simulink model "Appl_DrMemory_CtrlModel"  (R2018b)
settings: configuration reference "CodeConfig_10_ms" (kept outside this file)
undefined symbols (not defined in the file): CAL_DrMem_100MS, CAL_DrMem_90MS, D_DRMEM_SPEED_5, D_ToleranceDistance, FALSE, TRUE
libraries: DareLib x92, simulink x1
(part 3 of 3)

== stateflow chart Appl_DrMemory_CtrlModel/UpDataInputInfo/InputSignalProcess/MemorySetCallPreconditionDeal/PreconditionDeal ==
  state MemorySetPreconditionDeal [parallel]
    settings: executionOrder=1
    state PreconditionSatisfied
      en:
      MemSetPC_Flag = TRUE;
    state PreconditionNotSatisfied
      en:
      MemSetPC_Flag = FALSE;
    (default) -> MemorySetPreconditionDeal.PreconditionNotSatisfied
    MemorySetPreconditionDeal.PreconditionNotSatisfied -> MemorySetPreconditionDeal.PreconditionSatisfied : /*调节配置 == 1six way motor ||  2 twelve way motor
        | && 记忆功能使能 == 0x1:TRUE
        | && 座椅已学习
        | && 座椅运动类型 == 0x0:enNULL
        | && 座椅霍尔故障标志位 == FALSE
        | && 座椅继电器粘连故障标志位 == FALSE
        | && 座椅堵转故障标志位 == FALSE
        | && IVI_NapMode_SwtichSet != 0x1:打开小憩模式
        | && 电压模式 == 正常
        | && DrMem_NapMode != enNapMode.EN_NapMode_Open...
        | /PreMemSetStop = 0x0:enNone;*/
        | [(DrMem_AdjustEnable == 1 || DrMem_AdjustEnable == 2) ...
        | && DrMem_MemoryConfig == TRUE ...
        | && DrMem_SeatLearnResult == TRUE ...
        | && DrMem_CurrentMoveType == enSeatMotorRunType.EN_NULL ...
        | && DrMem_AnyoneHallFaultSts == FALSE ...
        | && DrMem_AnyoneRelayFaultSts == FALSE ...
        | && DrMem_AnyoneLockFaultSts == FALSE ...
        | && DrMem_VoltSatisfy == TRUE ...
        | && DrMem_VoltMode == enFinalPowerMode.EN_NORMAL_VOLT]
        | /PreMemSetStop = enMemStopCause.EN_MemStop_NULL;
    MemorySetPreconditionDeal.PreconditionSatisfied -> MemorySetPreconditionDeal.PreconditionNotSatisfied [order 1] : /*记忆功能使能 != 0x1:TRUE
        | /PreMemCallStop = 0xA:enConfigError;*/
        | [(DrMem_AdjustEnable != 1 && DrMem_AdjustEnable != 2) || DrMem_MemoryConfig != TRUE]
        | /PreMemSetStop = enMemStopCause.EN_MemStop_ConfigError;
    MemorySetPreconditionDeal.PreconditionSatisfied -> MemorySetPreconditionDeal.PreconditionNotSatisfied [order 2] : /*!座椅已学习
        | /PreMemSetStop = 0x1:enNotLearn;*/
        | [DrMem_SeatLearnResult != TRUE]
        | /PreMemSetStop = enMemStopCause.EN_MemStop_Learn;
    MemorySetPreconditionDeal.PreconditionSatisfied -> MemorySetPreconditionDeal.PreconditionNotSatisfied [order 3] : /*座椅运动类型 != 0x0:enNULL
        | /PreMemSetStop = 0x2:enOtherMove;*/
        | [DrMem_CurrentMoveType != enSeatMotorRunType.EN_NULL]
        | /PreMemSetStop = enMemStopCause.EN_MemStop_OtherMove;
    MemorySetPreconditionDeal.PreconditionSatisfied -> MemorySetPreconditionDeal.PreconditionNotSatisfied [order 4] : /*座椅霍尔故障标志位 != FALSE
        | /PreMemSetStop = 0x3:enHallError;*/
        | [DrMem_AnyoneHallFaultSts != FALSE]
        | /PreMemSetStop = enMemStopCause.EN_MemStop_HallErr;
    MemorySetPreconditionDeal.PreconditionSatisfied -> MemorySetPreconditionDeal.PreconditionNotSatisfied [order 5] : /*座椅继电器粘连故障标志位 != FALSE
        | /PreMemSetStop = 0x4:enRelayError;*/
        | [DrMem_AnyoneRelayFaultSts != FALSE]
        | /PreMemSetStop = enMemStopCause.EN_MemStop_RelayErr;
    MemorySetPreconditionDeal.PreconditionSatisfied -> MemorySetPreconditionDeal.PreconditionNotSatisfied [commented out] : /*IVI_NapMode_SwtichSet == 0x1:打开小憩模式
        | /PreMemSetStop = 0xB:enNapError;*/
        | [DrMem_NapMode == enNapMode.EN_NapMode_Open]
        | /PreMemSetStop = enMemStopCause.EN_MemStop_NapError;
    MemorySetPreconditionDeal.PreconditionSatisfied -> MemorySetPreconditionDeal.PreconditionNotSatisfied [order 7] : /*座椅堵转故障标志位 != FALSE
        | /PreMemSetStop = 0x5:EN_MemStop_StallErr(;*/
        | [DrMem_AnyoneLockFaultSts != FALSE]
        | /PreMemSetStop = enMemStopCause.EN_MemStop_StallErr;
    MemorySetPreconditionDeal.PreconditionSatisfied -> MemorySetPreconditionDeal.PreconditionNotSatisfied [order 6] : /*电压模式 != 正常
        | /PreMemSetStop = 0xE:enVoltageError;*/
        | [DrMem_VoltMode != enFinalPowerMode.EN_NORMAL_VOLT || TRUE != DrMem_VoltSatisfy]
        | /PreMemSetStop = enMemStopCause.EN_MemStop_VoltageErr;
  state MemoryCallPreconditionDeal [parallel]
    settings: executionOrder=2
    state PreconditionSatisfied
      en:
      MemCallPC_Flag = TRUE;
    state PreconditionNotSatisfied
      en:
      MemCallPC_Flag = FALSE;
    (default) -> MemoryCallPreconditionDeal.PreconditionNotSatisfied
    MemoryCallPreconditionDeal.PreconditionNotSatisfied -> MemoryCallPreconditionDeal.PreconditionSatisfied : /*调节配置 == 1six way motor ||  2 twelve way motor
        | &&记忆功能使能 == 0x1:TRUE
        | && 电源档位 != 0x3:enCRANK
        | && GearPN_Flag == TRUE
        | && 座椅已学习
        | && 座椅继电器粘连故障标志位 == FALSE
        | && SpeedLessThan5_Flag == TRUE
        | && 座椅运动类型 <= 0x3:enMemory
        | && 电压模式 == 正常
        | && 座椅按键标志位 == FALSE
        | && DSM_NapMode_FB != 0x2:打开小憩模式
        | /PreMemCallStop = 0x0:enNone;*/
        | [(DrMem_AdjustEnable == 1 || DrMem_AdjustEnable == 2) ...
        | && DrMem_MemoryConfig == TRUE ...
        | && DrMem_PowerMode != enPowerModeSts.EN_CRANK ...
        | && DrMem_Gear_PN_FlagOut == TRUE ...
        | && DrMem_SeatLearnResult == TRUE ...
        | && DrMem_AnyoneRelayFaultSts == FALSE ...
        | && SpeedLessThan5_Flag == TRUE ...
        | && DrMem_HeightSwitch == FALSE ...
        | && DrMem_LengthSwitch == FALSE ...
        | && DrMem_BackSwitch == FALSE ...
        | && (DrMem_FrontSwitch == FALSE || DrMem_AdjustEnable == 1) ...
        | && DrMem_CurrentMoveType <= enSeatMotorRunType.EN_MemoryEnable ...
        | && DrMem_VoltSatisfy == TRUE...
        | && DrMem_VoltMode == enFinalPowerMode.EN_NORMAL_VOLT ...
        | && DrMem_NapMode != enNapMode.EN_NapMode_Open]
        | /PreMemCallStop = enMemStopCause.EN_MemStop_NULL;
    MemoryCallPreconditionDeal.PreconditionSatisfied -> MemoryCallPreconditionDeal.PreconditionNotSatisfied [order 1] : /*记忆功能使能 != 0x1:TRUE
        | /PreMemCallStop = 0xA:enConfigError;*/
        | [(DrMem_AdjustEnable != 1 && DrMem_AdjustEnable != 2) || DrMem_MemoryConfig != TRUE]
        | /PreMemCallStop = enMemStopCause.EN_MemStop_ConfigError;
    MemoryCallPreconditionDeal.PreconditionSatisfied -> MemoryCallPreconditionDeal.PreconditionNotSatisfied [order 7] : /*电源档位 == 0x3:enCRANK
        | /PreMemCallStop = 0x6:enNotON;*/
        | [DrMem_PowerMode == enPowerModeSts.EN_CRANK]
        | /PreMemCallStop = enMemStopCause.EN_MemStop_NotON;
    MemoryCallPreconditionDeal.PreconditionSatisfied -> MemoryCallPreconditionDeal.PreconditionNotSatisfied [order 8] : /*GearPN_Flag != TRUE
        | /PreMemCallStop = 0x7:enNotGearPN;*/
        | [DrMem_Gear_PN_FlagOut != TRUE]
        | /PreMemCallStop = enMemStopCause.EN_MemStop_NotGearPN;
    MemoryCallPreconditionDeal.PreconditionSatisfied -> MemoryCallPreconditionDeal.PreconditionNotSatisfied [order 2] : /*!座椅已学习
        | /PreMemSetStop = 0x1:enNotLearn;*/
        | [DrMem_SeatLearnResult != TRUE]
        | /PreMemCallStop = enMemStopCause.EN_MemStop_Learn;
    MemoryCallPreconditionDeal.PreconditionSatisfied -> MemoryCallPreconditionDeal.PreconditionNotSatisfied [order 4] : /*座椅继电器粘连故障标志位 != FALSE
        | /PreMemSetStop = 0x4:enRelayError;*/
        | [DrMem_AnyoneRelayFaultSts != FALSE]
        | /PreMemCallStop = enMemStopCause.EN_MemStop_RelayErr;
    MemoryCallPreconditionDeal.PreconditionSatisfied -> MemoryCallPreconditionDeal.PreconditionNotSatisfied [order 9] : /*SpeedLessThan5_Flag != TRUE
        | /PreMemCallStop = 0x8:enSpeedError;*/
        | [SpeedLessThan5_Flag != TRUE]
        | /PreMemCallStop = enMemStopCause.EN_MemStop_SpeedError;
    MemoryCallPreconditionDeal.PreconditionSatisfied -> MemoryCallPreconditionDeal.PreconditionNotSatisfied [order 3] : /*座椅运动类型 > 0x3:enMemory
        | /PreMemCallStop = 0x2:enOtherMove;*/
        | [DrMem_CurrentMoveType > enSeatMotorRunType.EN_MemoryEnable]
        | /PreMemCallStop = enMemStopCause.EN_MemStop_OtherMove;
    MemoryCallPreconditionDeal.PreconditionSatisfied -> MemoryCallPreconditionDeal.PreconditionNotSatisfied [order 5] : /*IVI_NapMode_SwtichSet == 0x1:打开小憩模式
        | /PreMemSetStop = 0xB:enNapError;*/
        | [DrMem_NapMode == enNapMode.EN_NapMode_Open]
        | /PreMemCallStop = enMemStopCause.EN_MemStop_NapError;
    MemoryCallPreconditionDeal.PreconditionSatisfied -> MemoryCallPreconditionDeal.PreconditionNotSatisfied [order 6] : /*电压模式 != 正常
        | /PreMemSetStop = 0xE:enVoltageError;*/
        | [DrMem_VoltMode != enFinalPowerMode.EN_NORMAL_VOLT || TRUE != DrMem_VoltSatisfy]
        | /PreMemCallStop = enMemStopCause.EN_MemStop_VoltageErr;
    MemoryCallPreconditionDeal.PreconditionSatisfied -> MemoryCallPreconditionDeal.PreconditionNotSatisfied [order 10] : /*按键状态 != FALSE
        | /PreMemSetStop = 0x5:EN_MemStop_StallErr(;*/
        | [DrMem_HeightSwitch != FALSE ...
        | || DrMem_LengthSwitch != FALSE ...
        | || DrMem_BackSwitch != FALSE ...
        | || (DrMem_FrontSwitch != FALSE && DrMem_AdjustEnable == 2)]
        | /PreMemCallStop = enMemStopCause.EN_MemStop_StallErr;
  data: FALSE parameter; TRUE parameter; DrMem_Gear_PN_FlagOut input; DrMem_PowerMode input; DrMem_VoltMode input; DrMem_AdjustEnable input; DrMem_AnyoneHallFaultSts input; DrMem_AnyoneRelayFaultSts input; DrMem_CurrentMoveType input; DrMem_SeatLearnResult input; DrMem_NapMode input; SpeedLessThan5_Flag input; MemSetPC_Flag output uint8; PreMemSetStop output Enum: enMemStopCause; MemCallPC_Flag output uint8; PreMemCallStop output Enum: enMemStopCause; DrMem_MemoryConfig input; DrMem_AnyoneLockFaultSts input; DrMem_VoltSatisfy input; DrMem_HeightSwitch input; DrMem_LengthSwitch input; DrMem_BackSwitch input; DrMem_FrontSwitch input

== stateflow chart Appl_DrMemory_CtrlModel/LogicCtrl/LocalAdjustCtrl/MemoryCall ==
  state MemoryCallLogic [parallel]
    settings: executionOrder=1
    state MemoryCallInactive
      en:
      MemoryCallFbSts = enMemCallFb.EN_MemCallFb_NULL;
      MemoryButtonNum = 0;
      MsgSendFinishedFlag = FALSE;
      SeatMemoryValidReq = FALSE;
      SeatHeightPosiReq = 0;
      SeatLengthPosiReq = 0;
      SeatBackPosiReq = 0;
      SeatFrontPosiReq = 0;
    state MemoryCallActive
      state Wait
        (default) -> (junction 52)
        Wait -> (junction 52) [order 1]
        (junction 52) -> (junction 55)
        (junction 55) -> (junction 57) [order 1] : /*获取记忆调用1目标位置*/
            | [SeatMemBtn == enMemBtn.EN_MemBtn_Call1]
        (junction 55) -> (junction 63) [order 2]
        (junction 57) -> (junction 59) : {MemoryButtonNum = 1;
            | SeatMemoryValidReq = MemoryValid;
            | SeatHeightPosiReq = MemoryHeightPosi;
            | SeatLengthPosiReq = MemoryLengthPosi;
            | SeatBackPosiReq = MemoryBackPosi;
            | SeatFrontPosiReq = MemoryFrontPosi;}
        (junction 59) -> (junction 63)
        (junction 63) -> (junction 67)
        (junction 67) -> (junction 69) [order 1] : /*获取记忆调用2目标位置*/
            | [SeatMemBtn == enMemBtn.EN_MemBtn_Call2]
        (junction 67) -> (junction 73) [order 2]
        (junction 69) -> (junction 71) : {MemoryButtonNum = 2;
            | SeatMemoryValidReq = MemoryValid;
            | SeatHeightPosiReq = MemoryHeightPosi;
            | SeatLengthPosiReq = MemoryLengthPosi;
            | SeatBackPosiReq = MemoryBackPosi;
            | SeatFrontPosiReq = MemoryFrontPosi;}
        (junction 71) -> (junction 73)
        (junction 73) -> (junction 76)
        (junction 76) -> (junction 78) [order 1] : /*获取记忆调用3目标位置*/
            | [SeatMemBtn == enMemBtn.EN_MemBtn_Call3]
        (junction 76) -> (junction 82) [order 2]
        (junction 78) -> (junction 80) : {MemoryButtonNum = 3;
            | SeatMemoryValidReq = MemoryValid;
            | SeatHeightPosiReq = MemoryHeightPosi;
            | SeatLengthPosiReq = MemoryLengthPosi;
            | SeatBackPosiReq = MemoryBackPosi;
            | SeatFrontPosiReq = MemoryFrontPosi;}
        (junction 80) -> (junction 82)
        (junction 82) -> (junction 85)
        (junction 85) -> (junction 126) [order 1] : /* 调用不满足 停止电机运动 */
            | [MemCallPC_Flag == FALSE || SeatMemoryValidReq == FALSE]
        (junction 85) -> (junction 131) [order 2] : {MemoryCallFbSts = enMemCallFb.EN_MemCallFb_Wait;}
        (junction 126) -> (junction 128) : {SeatMemoryValidReq = FALSE;
            | SeatHeightPosiReq = 0;
            | SeatLengthPosiReq = 0;
            | SeatBackPosiReq = 0;
            | SeatFrontPosiReq = 0;}
        (junction 128) -> (junction 131)
        (junction 131) -> (junction 133)
      state Succeed
        en:
        MemoryCallFbSts = enMemCallFb.EN_MemCallFb_Succeed;
        WaitTimeCnt = 0;
        //SetCanSendEvent();
        du:
        WaitTimeCnt += 1;
      state Fail
        en:
        MemoryCallFbSts = enMemCallFb.EN_MemCallFb_Faild;
        WaitTimeCnt = 0;
        //SetCanSendEvent();
        du:
        WaitTimeCnt += 1;
      state MessageSendFinish
        en:
        MsgSendFinishedFlag = TRUE;
        MemoryCallFbSts = enMemCallFb.EN_MemCallFb_NULL;
      note: /*如果服务层没有CAN反馈标志，使用延时90ms(20ms/5帧)*/
      (default) -> Wait
      Wait -> Succeed [order 4] : /*(高度自动运行成功标志位 == TRUE || 高度堵转)
          | && (纵向自动运行成功标志位 == TRUE || 纵向堵转)
          | && (靠背自动运行成功标志位 == TRUE || 靠背堵转)
          | && (前部自动运行成功标志位 == TRUE || 前部堵转)*/
          | [(DrMem_HeightAutoRunFlag == enSeatAutoRunSts.EN_SEAT_SUCCESS ...
          | || DrMem_HeightLockFault == TRUE) ...
          | && (DrMem_LengthAutoRunFlag == enSeatAutoRunSts.EN_SEAT_SUCCESS ...
          |     || DrMem_LengthLockFault == TRUE) ...
          | && (DrMem_BackAutoRunFlag == enSeatAutoRunSts.EN_SEAT_SUCCESS ...
          |     || DrMem_BackLockFault == TRUE) ...
          | && (DrMem_FrontAutoRunFlag == enSeatAutoRunSts.EN_SEAT_SUCCESS ...
          |     || DrMem_FrontLockFault == TRUE)]
      Wait -> MessageSendFinish [order 2] : /* 位置未记忆 */
          | [SeatMemoryValidReq == FALSE]
          | /MemCallStopReason = enMemStopCause.EN_MemStop_PosiError;
      Wait -> Fail [order 1] : /*记忆调用前置条件不满足*/
          | [MemCallPC_Flag == FALSE]
          | /MemCallStopReason = PreMemCallStop;
      Wait -> Fail [order 3] : /*1.此处接口需要与调节模型确认返回值
          | 2.此跳转包含霍尔故障
          | 高度自动运行成功标志位 == FALSE
          | || 纵向自动运行成功标志位 == FALSE
          | || 靠背自动运行成功标志位 == FALSE
          | || 前部自动运行成功标志位 == FALSE
          | /MemCallStopReason = 0xC:enMotorRunError*/
          | [DrMem_HeightAutoRunFlag == enSeatAutoRunSts.EN_SEAT_FAIL ...
          | || DrMem_LengthAutoRunFlag == enSeatAutoRunSts.EN_SEAT_FAIL ...
          | || DrMem_BackAutoRunFlag == enSeatAutoRunSts.EN_SEAT_FAIL ...
          | || DrMem_FrontAutoRunFlag == enSeatAutoRunSts.EN_SEAT_FAIL]
          | /MemCallStopReason = enMemStopCause.EN_MemStop_MotorRunErr;
      Succeed -> MessageSendFinish : /*Srvl_CAN反馈报文发送完成 || 延时90ms*/
          | [WaitTimeCnt >= 2 ...
          | && GetCanSendEvent() == TRUE]
      Fail -> MessageSendFinish : /*Srvl_CAN反馈报文发送完成 || 延时90ms*/
          | [WaitTimeCnt >= 2 ...
          | && GetCanSendEvent() == TRUE]
    (default) -> MemoryCallInactive
    MemoryCallInactive -> MemoryCallActive [order 1] : /*SeatMemBtn变为CallButton1*/
        | [hasChangedTo(SeatMemBtn,enMemBtn.EN_MemBtn_Call1)]
    MemoryCallInactive -> MemoryCallActive [order 2] : /*SeatMemBtn变为CallButton2*/
        | [hasChangedTo(SeatMemBtn,enMemBtn.EN_MemBtn_Call2)]
    MemoryCallInactive -> MemoryCallActive [order 3] : /*SeatMemBtn变为CallButton3*/
        | [hasChangedTo(SeatMemBtn,enMemBtn.EN_MemBtn_Call3)]
    MemoryCallActive -> MemoryCallInactive : [MsgSendFinishedFlag == TRUE]
  state [CallFB1,CallFB2,CallFB3] = MemCallWaitFBFunc(ButtonNum,FBSts) [function]
  state MemoryCallMessageFeedback [parallel]
    settings: executionOrder=2
    state MemoryCallDefaultFeedback
      en:
      SeatMem1StsFb = enMemCallFb.EN_MemCallFb_NULL;
      SeatMem2StsFb = enMemCallFb.EN_MemCallFb_NULL;
      SeatMem3StsFb = enMemCallFb.EN_MemCallFb_NULL;
    state MemoryCallResultFeedback
      state MemoryCallRun
        en:
        [SeatMem1StsFb,SeatMem2StsFb,SeatMem3StsFb] = MemCallWaitFBFunc(MemoryButtonNum,MemoryCallFbSts);
        du:
        [SeatMem1StsFb,SeatMem2StsFb,SeatMem3StsFb] = MemCallWaitFBFunc(MemoryButtonNum,MemoryCallFbSts);
      state MemoryCallMotorStop
        en:
        FbWaitTimeCnt = 0;
        [SeatMem1StsFb,SeatMem2StsFb,SeatMem3StsFb] = MemCallWaitFBFunc(MemoryButtonNum,MemoryCallFbSts);
        SetCanMemCall1(SeatMem1StsFb);
        SetCanMemCall2(SeatMem2StsFb);
        SetCanMemCall3(SeatMem3StsFb);
        SetCanSendEvent();
        du:
        FbWaitTimeCnt += 1;
      (default) -> MemoryCallRun
      MemoryCallRun -> MemoryCallMotorStop : /*记忆调用结束*/
          | [MemoryCallFbSts == enMemCallFb.EN_MemCallFb_Succeed ...
          | || MemoryCallFbSts == enMemCallFb.EN_MemCallFb_Faild]
    (default) -> MemoryCallDefaultFeedback
    MemoryCallDefaultFeedback -> MemoryCallResultFeedback [order 1] : /*记忆调用开始运行*/
        | [MemoryCallFbSts == enMemCallFb.EN_MemCallFb_Wait]
    MemoryCallDefaultFeedback -> MemoryCallMotorStop [order 2] : /*记忆调用直接结束*/
        | [MemoryCallFbSts == enMemCallFb.EN_MemCallFb_Succeed ...
        | || MemoryCallFbSts == enMemCallFb.EN_MemCallFb_Faild]
    MemoryCallMotorStop -> MemoryCallDefaultFeedback : /*1延时90ms*/
        | [FbWaitTimeCnt >= CAL_DrMem_90MS ...
        | || GetCanSendEvent() == TRUE]
  state SetCanSendEvent [function]
  state SetCanMemCall1(In1) [function]
  state SetCanMemCall2(In1) [function]
  state Out1 = GetCanSendEvent [function]
  state SetCanMemCall3(In1) [function]
  data: ButtonNum function_input; FBSts function_input; CallFB1 function_output; CallFB2 function_output; CallFB3 function_output; In1 function_input; In1 function_input; Out1 function_output; In1 function_input; SeatMemoryValidReq output uint8; SeatHeightPosiReq output uint16; SeatLengthPosiReq output uint16; SeatBackPosiReq output uint16; SeatFrontPosiReq output uint16; MemCallStopReason output Enum: enMemStopCause; MemoryCallFbSts local Enum: enMemCallFb; MemoryButtonNum local Enum: enMemCallFb; MsgSendFinishedFlag local uint8; FALSE parameter; SeatMemBtn input; MemoryHeightPosi input; MemoryLengthPosi input; MemoryBackPosi input; MemoryFrontPosi input; MemoryValid input; PreMemCallStop input; DrMem_HeightAutoRunFlag input; DrMem_LengthAutoRunFlag input; DrMem_BackAutoRunFlag input; DrMem_FrontAutoRunFlag input; TRUE parameter; WaitTimeCnt local uint16; CAL_DrMem_90MS parameter; MemCallPC_Flag input; DrMem_HeightLockFault input; DrMem_LengthLockFault input; DrMem_BackLockFault input; DrMem_FrontLockFault input; SeatMem1StsFb output Enum: enMemCallFb; SeatMem2StsFb output Enum: enMemCallFb; SeatMem3StsFb output Enum: enMemCallFb; FbWaitTimeCnt local uint16

== stateflow chart Appl_DrMemory_CtrlModel/LogicCtrl/LocalAdjustCtrl/MemorySetLogic/FirstPosiMemSetFunc/FirstPosiMemSetFunc ==
  state MemoryHight(CurrentH) [function]
  state MemoryLength(CurrentL) [function]
  state MemoryBack(CurrentB) [function]
  state MemoryFront(CurrentF) [function]
  state MemoryValid(Sts) [function]
  (default) -> (junction 2)
  (junction 2) -> (junction 10)
  (junction 10) -> (junction 12) [order 1] : /* 记忆功能使能 */
      | [SeatMemCfg == 1 || SeatMemCfg == 2]
  (junction 10) -> (junction 16) [order 2]
  (junction 12) -> (junction 14) : {MemoryHight(CurrentH);
      | MemoryLength(CurrentL);
      | MemoryBack(CurrentB);
      | MemoryFront(CurrentF);
      | MemoryValid(TRUE);}
  (junction 14) -> (junction 16)
  (junction 16) -> (junction 19)
  data: CurrentH function_input; CurrentL function_input; CurrentB function_input; CurrentF function_input; Sts function_input; SeatMemCfg input uint8; CurrentH input uint16; CurrentL input uint16; CurrentB input uint16; CurrentF input uint16; TRUE parameter

== stateflow chart Appl_DrMemory_CtrlModel/LogicCtrl/LocalAdjustCtrl/MemorySetLogic/SecondPosiMemSetFunc/SecondPosiMemSetFunc ==
  state MemoryHight(CurrentH) [function]
  state MemoryLength(CurrentL) [function]
  state MemoryBack(CurrentB) [function]
  state MemoryFront(CurrentF) [function]
  state MemoryValid(Sts) [function]
  (default) -> (junction 2)
  (junction 2) -> (junction 10)
  (junction 10) -> (junction 12) [order 1] : /* 记忆功能使能 */
      | [SeatMemCfg == 1 || SeatMemCfg == 2]
  (junction 10) -> (junction 16) [order 2]
  (junction 12) -> (junction 14) : {MemoryHight(CurrentH);
      | MemoryLength(CurrentL);
      | MemoryBack(CurrentB);
      | MemoryFront(CurrentF);
      | MemoryValid(TRUE);}
  (junction 14) -> (junction 16)
  (junction 16) -> (junction 19)
  data: CurrentH function_input; CurrentL function_input; CurrentB function_input; CurrentF function_input; Sts function_input; SeatMemCfg input uint8; CurrentH input uint16; CurrentL input uint16; CurrentB input uint16; CurrentF input uint16; TRUE parameter

== stateflow chart Appl_DrMemory_CtrlModel/UpDataInputInfo/InputSignalProcess/VehicleSpeedDeal/SpeedDeal ==
  state MoreThan5
    en:
    SpeedLessThan5_Flag = FALSE;
  state LessThan5
    en:
    SpeedLessThan5_Flag = TRUE;
  (default) -> MoreThan5
  LessThan5 -> MoreThan5 : /*ABS报文不在线
      | || 车速信号有效性 != 0x0:valid
      | || 车速 > D_5km_per_hour*/
      | [DrMem_0x284_SpeedLostFlag == TRUE ...
      | || DrMem_VehicleSpeedValid != FALSE...
      | || DrMem_VehicleSpeed > D_DRMEM_SPEED_5]
  MoreThan5 -> LessThan5 : /*ABS报文在线
      | && 车速信号有效性 == 0x0:valid
      | && 车速 ≤ D_5km_per_hour*/
      | [DrMem_0x284_SpeedLostFlag == FALSE ...
      | && DrMem_VehicleSpeedValid == FALSE...
      | && DrMem_VehicleSpeed <= D_DRMEM_SPEED_5]
  data: TRUE parameter; FALSE parameter; DrMem_0x284_SpeedLostFlag input; DrMem_VehicleSpeedValid input; DrMem_VehicleSpeed input; SpeedLessThan5_Flag output uint8; D_DRMEM_SPEED_5 parameter

== stateflow chart Appl_DrMemory_CtrlModel/LogicCtrl/LocalAdjustCtrl/MemorySetLogic/ThirdPosiMemSetFunc/ThirdPosiMemSetFunc ==
  state MemoryHight(CurrentH) [function]
  state MemoryLength(CurrentL) [function]
  state MemoryBack(CurrentB) [function]
  state MemoryFront(CurrentF) [function]
  state MemoryValid(Sts) [function]
  (default) -> (junction 2)
  (junction 2) -> (junction 10)
  (junction 10) -> (junction 12) [order 1] : /* 记忆功能使能 */
      | [SeatMemCfg == 1 || SeatMemCfg == 2]
  (junction 10) -> (junction 16) [order 2]
  (junction 12) -> (junction 14) : {MemoryHight(CurrentH);
      | MemoryLength(CurrentL);
      | MemoryBack(CurrentB);
      | MemoryFront(CurrentF);
      | MemoryValid(TRUE);}
  (junction 14) -> (junction 16)
  (junction 16) -> (junction 19)
  data: CurrentH function_input; CurrentL function_input; CurrentB function_input; CurrentF function_input; Sts function_input; SeatMemCfg input uint8; CurrentH input uint16; CurrentL input uint16; CurrentB input uint16; CurrentF input uint16; TRUE parameter

== stateflow chart Appl_DrMemory_CtrlModel/LogicCtrl/LocalAdjustCtrl/MemoryCall/MemCallWaitFBFunc/Chart ==
  (default) -> (junction 3)
  (junction 3) -> (junction 5) : {CallFB1 = enMemCallFb.EN_MemCallFb_NULL;
      | CallFB2 = enMemCallFb.EN_MemCallFb_NULL;
      | CallFB3 = enMemCallFb.EN_MemCallFb_NULL;}
  (junction 5) -> (junction 7) [order 1] : /* 调用位置1进行中 */
      | [ButtonNum == 1]
  (junction 5) -> (junction 14) [order 2]
  (junction 7) -> (junction 9) : {CallFB1 = FBSts;}
  (junction 14) -> (junction 16) [order 1] : /* 调用位置2 进行中 */
      | [ButtonNum == 2]
  (junction 14) -> (junction 20) [order 2] : {CallFB3 = FBSts;}
  (junction 16) -> (junction 18) : {CallFB2 = FBSts;}
  (junction 18) -> (junction 20)
  (junction 9) -> (junction 18)
  (junction 20) -> (junction 27)
  data: ButtonNum input uint8; FBSts input Enum: enMemCallFb; CallFB1 output Enum: enMemCallFb; CallFB2 output Enum: enMemCallFb; CallFB3 output Enum: enMemCallFb
